simulink model "demomf"  (Simulink 6.2)
settings: Solver=ode45  StartTime=0.0  StopTime=200  FixedStep=0.1  RelTol=1e-3
libraries: simulink_extras x2, simulink x1, marine_gnc x1
settings Model: LastModifiedBy=perez
settings DataIOCC: SignalLoggingName=sigsOut
settings OptimizationCC: BooleanDataType=off  InlineInvariantSignals=on
settings HardwareCC: TargetUnknown=on
settings GRTTargetCC: ModelReferenceCompliant=off  MatFileLogging=off

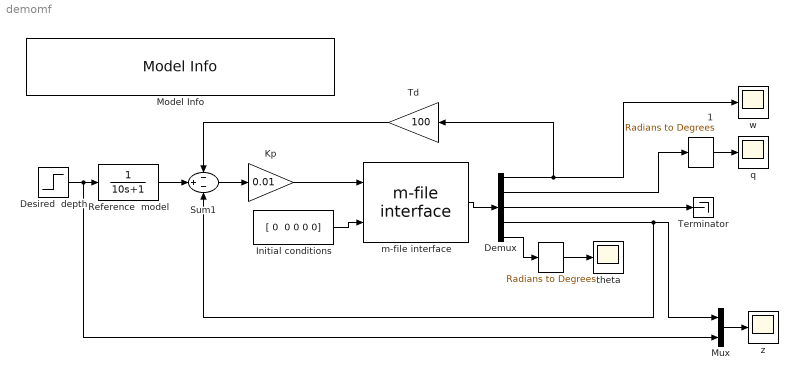
== system demomf ==
  "   " : simulink_extras/Transformations/Radians to Degrees
  "   1" : simulink_extras/Transformations/Radians to Degrees
  Demux : Demux  Outputs=5
  Desired  depth : Step  Time=30  After=50  SampleTime=0
  Initial conditions : Constant  Value="[ 0  0 0 0 0]"
  Kp : Gain  Gain=0.01  SaturateOnIntegerOverflow=on
  Model Info : simulink/Model-Wide Utilities/Model Info  InitialBlockCM=None  BlockCM=None  Frame=on  DisplayStringWithTags=|  HorizontalTextAlignment=Left  LeftAlignmentValue=0.02  SourceBlockDiagram=demomf  TagMaxNumber=20
      | Deep submergence rescue vehicle (DSRV) depth control system
      | Simulink interface to the GNC Toolbox m-file vessel models
      | %<Creator>Author: Thor I. Fossen
      | %<LastModificationDate>
  Mux : Mux  Inputs=2
  Reference  model : TransferFcn  Denominator=[10 1]
  Sum1 : Sum  Inputs=-+-  SaturateOnIntegerOverflow=on  InputSameDT=on
  Td : Gain  Orientation=left  Gain=100  SaturateOnIntegerOverflow=on
  Terminator : Terminator
  m-file interface : marine_gnc/Examples/Vessels/m-file interface  vessmodel=DSRV  dimu_model=1  dimx_model=5
  q : Scope
      settings: TimeRange=200  YMin=-1.5  YMax=0.5
  theta : Scope
      settings: TimeRange=200  YMin=-8  YMax=0  SaveName=ScopeData4
  w : Scope
      settings: TimeRange=200  YMin=0  YMax=0.2  SaveName=ScopeData3
  z : Scope
      settings: TimeRange=200  YMin=0  YMax=80
  wires:
  Initial conditions/1 -> m-file interface/2
  m-file interface/1 -> Demux/1
  Demux/1 -> w/1, Td/1
  Demux/2 -> "   1"/1
  Kp/1 -> m-file interface/1
  Desired  depth/1 -> Reference  model/1, Mux/2
  Reference  model/1 -> Sum1/2
  Sum1/1 -> Kp/1
  Td/1 -> Sum1/1
  "   "/1 -> theta/1
  "   1"/1 -> q/1
  Mux/1 -> z/1
  Demux/4 -> Sum1/3, Mux/1
  Demux/3 -> Terminator/1
  Demux/5 -> "   "/1
